simulink model "Fahrrad2"  (Simulink 7.2)
settings: Solver=ode3  StartTime=0.0  StopTime=100.00  FixedStep=0.01  RelTol=1e-3
values from neighbouring files (symbols this model uses):
  dmv = d*1*v    (= 1.8)    [koeff.m]
  h2mg = h/2*m*g    (= 242.7975)    [koeff.m]
  J = bm*h*h    (= 4.05)    [koeff.m]
  Jsh2m = Js + h*h*m    (= 57.05)    [koeff.m]
  Kd = [0.00001 0.00001]    [koeff.m]
  Ki = [0.05 0.05]    [koeff.m]
  Kp = [0.005 0.005]    [koeff.m]
  mhg = 1 / (m*h*g)    (= 0.00205932927645)    [koeff.m]
  mv2 = m * v * v    (= 495)    [koeff.m]
  tau = 0.01    [koeff.m]
  v = 3    [koeff.m]
libraries: simulink x1
settings Model: Creator=Markus  LastModifiedBy=dpara
settings SolverCC: ZeroCrossAlgorithm=Adaptive
settings DebuggingCC: StrictBusMsg=ErrorLevel1

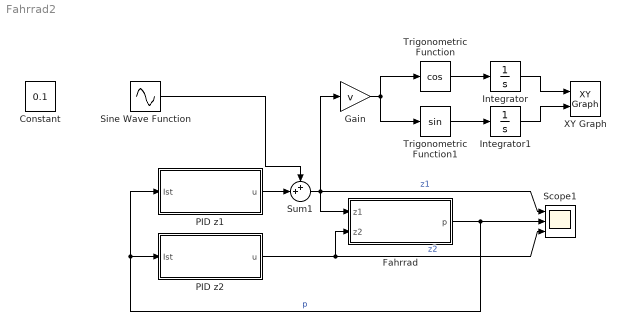
== system Fahrrad2 ==
  Constant : Constant  Value=0.1  OutDataType=sfix(16)  OutScaling=2^0
  Fahrrad : Subsystem
  Gain : Gain  Gain=v  ParameterDataType=sfix(16)  ParameterScaling=2^0  OutDataType=sfix(16)  OutScaling=2^0
  Integrator : Integrator
  Integrator1 : Integrator
  PID z1 : Subsystem  mask{i=1}
      mask prompts: i "Koeffizient index"
  PID z2 : Subsystem  mask{i=2}
      mask prompts: i "Koeffizient index"
  Scope1 : Scope  NumInputPorts=3
      settings: TimeRange=10  YMin=-0.03~-2~-0.1  YMax=0.05~2~0.1
  Sine Wave Function : Sin  Amplitude=0.05  Frequency=0.1  SampleTime=0
  Sum1 : Sum  Inputs=++|
  Trigonometric Function : Trigonometry  Operator=cos
  Trigonometric Function1 : Trigonometry
  XY Graph : simulink/Sinks/XY Graph  SystemSampleTime=-1  xmin=-10  xmax=100  ymin=-10  ymax=10  st=-1
  wires:
  Fahrrad/1(p) -> PID z1/1(Ist), PID z2/1(Ist), Scope1/2  "p"
  Gain/1 -> Trigonometric Function/1, Trigonometric Function1/1
  Trigonometric Function/1 -> Integrator/1
  Trigonometric Function1/1 -> Integrator1/1
  Integrator/1 -> XY Graph/1
  Integrator1/1 -> XY Graph/2
  PID z2/1(u) -> Fahrrad/2(z2), Scope1/3  "z2"
  Sum1/1 -> Fahrrad/1(z1), Gain/1, Scope1/1  "z1"
  PID z1/1(u) -> Sum1/2
  Sine Wave Function/1 -> Sum1/1

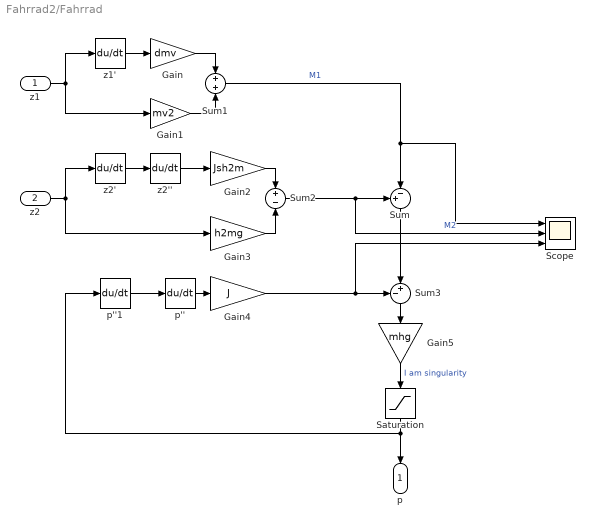
== system Fahrrad2/Fahrrad ==
  z1 : Inport
  z2 : Inport  Port=2
  Gain : Gain  Gain=dmv  ParameterDataType=sfix(16)  ParameterScaling=2^0  OutDataType=sfix(16)  OutScaling=2^0
  Gain1 : Gain  Gain=mv2  ParameterDataType=sfix(16)  ParameterScaling=2^0  OutDataType=sfix(16)  OutScaling=2^0
  Gain2 : Gain  Gain=Jsh2m  ParameterDataType=sfix(16)  ParameterScaling=2^0  OutDataType=sfix(16)  OutScaling=2^0
  Gain3 : Gain  Gain=h2mg  ParameterDataType=sfix(16)  ParameterScaling=2^0  OutDataType=sfix(16)  OutScaling=2^0
  Gain4 : Gain  Gain=J  ParameterDataType=sfix(16)  ParameterScaling=2^0  OutDataType=sfix(16)  OutScaling=2^0
  Gain5 : Gain  Orientation=down  Gain=mhg  ParameterDataType=sfix(16)  ParameterScaling=2^0  OutDataType=sfix(16)  OutScaling=2^0
  Saturation : Saturate  Orientation=down  UpperLimit=pi/2  LowerLimit=-pi/2  OutDataType=sfix(16)  OutScaling=2^0
  Scope : Scope  NumInputPorts=3
      settings: YMin=-0.5~3e-006~-0.0006  YMax=0.5~1.3e-005~0.0007
  Sum : Sum  Orientation=down  Inputs=+-|
  Sum1 : Sum  Inputs=+|+  OutDataType=sfix(16)  OutScaling=2^0
  Sum2 : Sum  Inputs=+|-  OutDataType=sfix(16)  OutScaling=2^0
  Sum3 : Sum  Orientation=down  Inputs=-+|
  p'' : Derivative
  p''1 : Derivative
  z1' : Derivative
  z2' : Derivative
  z2'' : Derivative
  p : Outport  Orientation=down
  wires:
  z1/1 -> z1'/1, Gain1/1
  z1'/1 -> Gain/1
  Gain1/1 -> Sum1/2
  Gain/1 -> Sum1/1
  Gain3/1 -> Sum2/2
  z2/1 -> z2'/1, Gain3/1
  z2'/1 -> z2''/1
  z2''/1 -> Gain2/1
  Gain2/1 -> Sum2/1
  p''/1 -> Gain4/1
  Sum1/1 -> Sum/2, Scope/1  "M1"
  Sum2/1 -> Sum/1, Scope/2  "M2"
  Sum/1 -> Sum3/2
  Gain4/1 -> Sum3/1, Scope/3
  Sum3/1 -> Gain5/1
  Gain5/1 -> Saturation/1  "I am singularity"
  p''1/1 -> p''/1
  Saturation/1 -> p/1, p''1/1

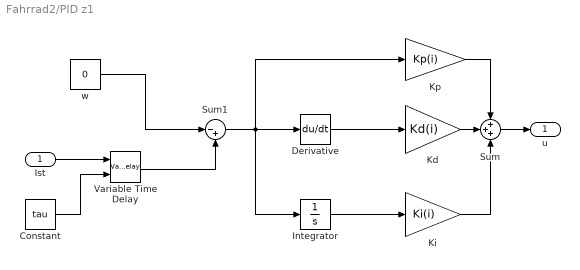
== system Fahrrad2/PID z1 ==
  Ist : Inport
  Constant : Constant  Value=tau
  Derivative : Derivative
  Integrator : Integrator
  Kd : Gain  Gain=Kd(i)
  Ki : Gain  Gain=Ki(i)
  Kp : Gain  Gain=Kp(i)
  Sum : Sum  Inputs=+++
  Sum1 : Sum  Inputs=|-+
  Variable Time Delay : VariableTransportDelay  MaximumDelay=10
  w : Constant  Value=0
  u : Outport
  wires:
  Kp/1 -> Sum/1
  Sum/1 -> u/1
  Ist/1 -> Variable Time Delay/1
  Constant/1 -> Variable Time Delay/2
  Integrator/1 -> Ki/1
  Derivative/1 -> Kd/1
  Kd/1 -> Sum/2
  Ki/1 -> Sum/3
  w/1 -> Sum1/1
  Variable Time Delay/1 -> Sum1/2
  Sum1/1 -> Derivative/1, Kp/1, Integrator/1

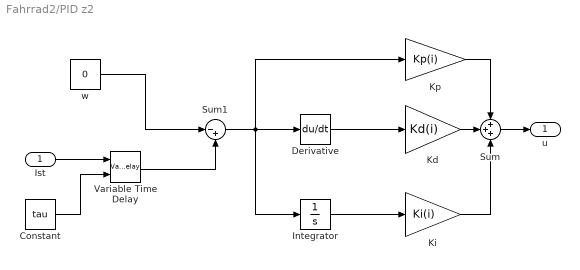
== system Fahrrad2/PID z2 ==
  Ist : Inport
  Constant : Constant  Value=tau
  Derivative : Derivative
  Integrator : Integrator
  Kd : Gain  Gain=Kd(i)
  Ki : Gain  Gain=Ki(i)
  Kp : Gain  Gain=Kp(i)
  Sum : Sum  Inputs=+++
  Sum1 : Sum  Inputs=|-+
  Variable Time Delay : VariableTransportDelay  MaximumDelay=10
  w : Constant  Value=0
  u : Outport
  wires:
  Sum1/1 -> Integrator/1, Kp/1, Derivative/1
  Variable Time Delay/1 -> Sum1/2
  w/1 -> Sum1/1
  Ki/1 -> Sum/3
  Kd/1 -> Sum/2
  Derivative/1 -> Kd/1
  Integrator/1 -> Ki/1
  Constant/1 -> Variable Time Delay/2
  Ist/1 -> Variable Time Delay/1
  Sum/1 -> u/1
  Kp/1 -> Sum/1
